simulink model "RC_proportionalcontrol"  (R2020a)
settings: Solver=VariableStepAuto  StartTime=0.0  StopTime=200  RelTol=1e-3
settings Model: Creator=Ulas  LastModifiedBy=Ulas

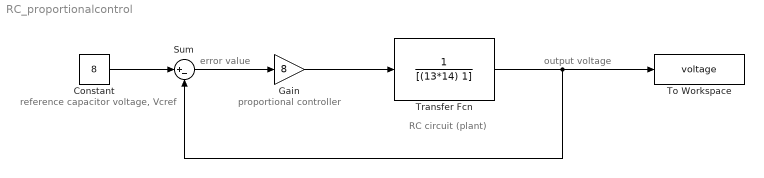
== system RC_proportionalcontrol ==
  note: reference capacitor voltage, Vcref
  note: error value
  note: RC circuit (plant)
  note: proportional controller
  note: output voltage
  Constant : Constant  Value=8
  Gain : Gain  Gain=8
  Sum : Sum  Inputs=|+-
  To Workspace : ToWorkspace  VariableName=voltage  SaveFormat=Timeseries  SampleTime=-1
  Transfer Fcn : TransferFcn  Denominator=[(13*14) 1]
  wires:
  Constant/1 -> Sum/1
  Sum/1 -> Gain/1
  Gain/1 -> Transfer Fcn/1
  Transfer Fcn/1 -> To Workspace/1, Sum/2
